simulink model "AM"  (R2020b)
settings: Solver=VariableStepAuto  StartTime=0.0  StopTime=1  RelTol=1e-3
undefined symbols (not defined in the file): magnitude
libraries: dsparch4 x2
settings Model: Creator=LENOVO  LastModifiedBy=LENOVO

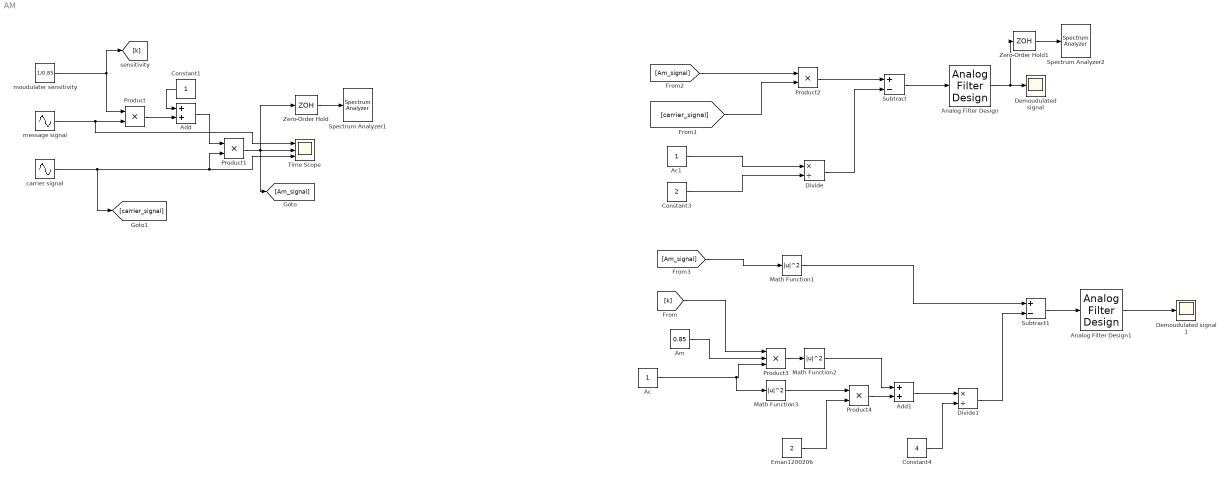
== system AM ==
  Ac : Constant
  Ac1 : Constant
  Add : Sum
  Add1 : Sum
  Am : Constant  Value=0.85
  Analog Filter Design : dsparch4/Analog Filter Design  method=Butterworth  filttype=Lowpass  N=2  Wlo=1000*2*pi  Whi=80  Rp=2  Rs=40
  Analog Filter Design1 : dsparch4/Analog Filter Design  method=Butterworth  filttype=Lowpass  N=2  Wlo=1000*2*pi  Whi=80  Rp=2  Rs=40
  Constant1 : Constant
  Constant3 : Constant  Value=2
  Constant4 : Constant  Value=4
  "Demoudulated signal " : Scope
  Demoudulated signal 1 : Scope
  Divide : Product  Inputs=*/
  Divide1 : Product  Inputs=*/
  Eman1200206 : Constant  Value=2
  Math Function1 : Math  Operator=magnitude^2  SaturateOnIntegerOverflow=on
  Math Function2 : Math  Operator=magnitude^2  SaturateOnIntegerOverflow=on
  Math Function3 : Math  Operator=magnitude^2  SaturateOnIntegerOverflow=on
  Product{,1..2,4} (4 alike) : Product
  Product3 : Product  Inputs=3
  Spectrum Analyzer1 : SpectrumAnalyzer
  Spectrum Analyzer2 : SpectrumAnalyzer
  Subtract : Sum  Inputs=+-
  Subtract1 : Sum  Inputs=+-
  Time Scope : Scope  NumInputPorts=3
  Zero-Order Hold : ZeroOrderHold  SampleTime=-1
  Zero-Order Hold1 : ZeroOrderHold  SampleTime=-1
  "carrier signal " : Sin  Frequency=2*pi*15000  Phase=90*2*pi  SampleTime=0
  message signal : Sin  Amplitude=0.85  Frequency=2*pi*1000  Phase=90*2*pi  SampleTime=0
  moudulater sensitivity : Constant  Value=1/0.85
  wires:
  moudulater sensitivity/1 -> Product/1, [k]
  Product/1 -> Add/2
  Constant1/1 -> Add/1
  Add/1 -> Product1/1
  "carrier signal "/1 -> Time Scope/3, Product1/2, [carrier_signal]
  [carrier_signal] -> Product2/2
  [Am_signal] -> Product2/1
  Product2/1 -> Subtract/1
  Ac1/1 -> Divide/1
  Constant3/1 -> Divide/2
  Divide/1 -> Subtract/2
  Subtract/1 -> Analog Filter Design/1
  Analog Filter Design/1 -> Zero-Order Hold1/1, "Demoudulated signal "/1
  [k] -> Product3/1
  Am/1 -> Product3/2
  Ac/1 -> Math Function3/1, Product3/3
  Analog Filter Design1/1 -> Demoudulated signal 1/1
  Subtract1/1 -> Analog Filter Design1/1
  Eman1200206/1 -> Product4/2
  Product4/1 -> Add1/2
  Constant4/1 -> Divide1/2
  Add1/1 -> Divide1/1
  Divide1/1 -> Subtract1/2
  Product3/1 -> Math Function2/1
  Math Function3/1 -> Product4/1
  Math Function2/1 -> Add1/1
  [Am_signal] -> Math Function1/1
  Math Function1/1 -> Subtract1/1
  Product1/1 -> [Am_signal], Zero-Order Hold/1, Time Scope/2
  message signal/1 -> Time Scope/1, Product/2
  Zero-Order Hold/1 -> Spectrum Analyzer1/1
  Zero-Order Hold1/1 -> Spectrum Analyzer2/1
